simulink model "EV_system"  (R2022b)
settings: Solver=VariableStepAuto  StartTime=0.0  StopTime=10  RelTol=1e-3
libraries: fl_lib x45, nesl_utility x31, ee_lib x16, simulink x2, sdl_lib x1
(part 1 of 2)
settings Model: Creator=guenk  LastModifiedBy=user
settings DebuggingCC: UnitsInconsistencyMsg=none

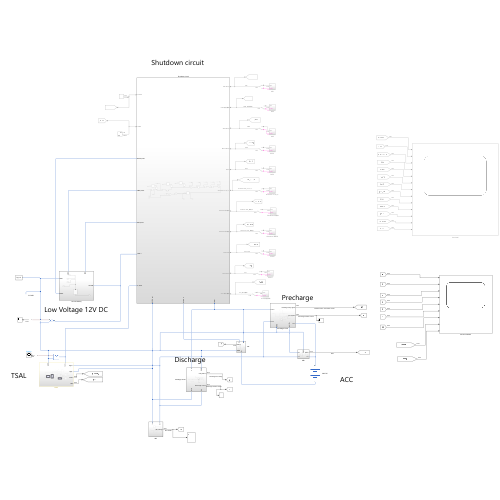
[thumbnail: Simulink's stored preview of the top-level diagram]
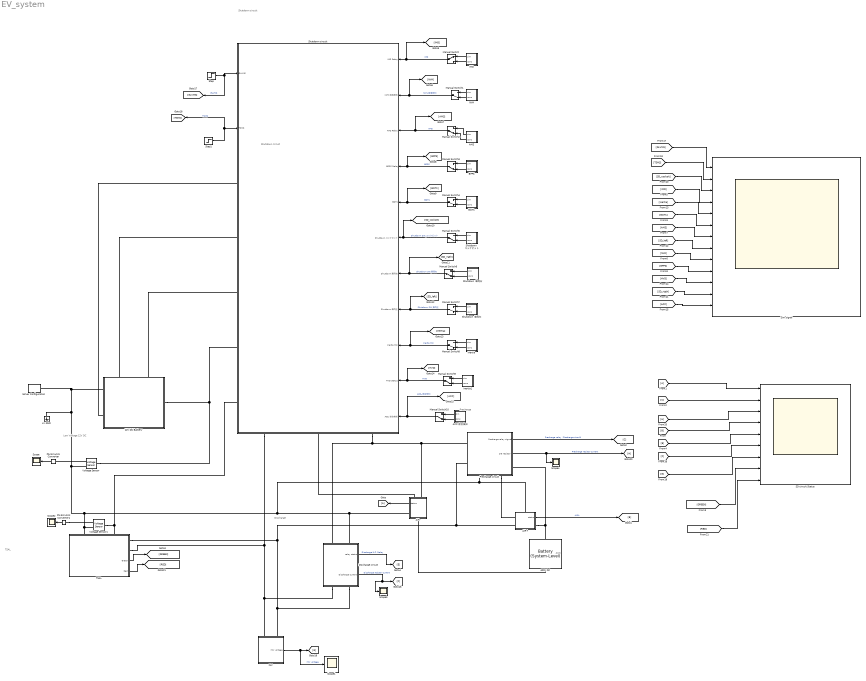
== system EV_system ==
  note: Precharge
  note: Discharge
  note: ACC
  note: Shutdown circuit
  note: Shutdown circuit
  note: Low Voltage 12V DC
  note: TSAL
  12V DC Battery : Subsystem
      settings: PortSchema="{\"entries\":[{\"content\":{\"sides\":[{\"content\":{\"connectorIds\":[\"LConn1\"]},\"type\":\"ConnectorPlacement.EquallySpacedRectSide\",\"uuid\":\"afe12baa-50eb-4c84-88de-44aa208358b8\"},{\"content\":{\"connectorIds\":[\"RConn1\",\"RConn2\"],\"side\":\"RIGHT\"},\"type\":\"ConnectorPlacement.EquallySpacedRectSide\",\"uuid\":\"76bb4b20-2fab-48ed-b43b-144bf9d425a6\"},{\"content\":{\"connectorIds\":[\"LConn2\",\"LConn3\"],\"side\":\"TOP\"},\"type\":\"ConnectorPlacement.EquallySpacedRectSide\",\"uuid\":\"9999fc27-06ad-4142-bc0d-dff183d80669\"},{\"content\":{\"connectorIds\":[],\"side\":\"BOTTOM\"},\"type\":\"ConnectorPlacement.EquallySpacedRectSide\",\"uuid\":\"0e91a3f8-fc00-4400-a4ba-be2b76be3e17\"}]},\"type\":\"ConnectorPlacement.EquallySpacedConnector\",\"uuid\":\"c30d57d7-3d09-4e60-950b-ccafea7457a0\"}],\"packageUris\":[\"http://schema.mathworks.com/mf0/Connector/R2020b\"],\"version\":\"1.0\"}"
  400V DC : sdl_lib/Sources/Battery (System-Level)  Vnom=400 V  R1=2 Ohm  prm_AH=sdl.enum.InfiniteFinite.Infinite  AH=50 A*hr  V1=11.5 V  AH1=25 A*hr  prm_R2=sdl.enum.DisabledEnabled.Disabled  R2=2000 Ohm  thermal_port=simscape.enum.thermaleffects.omit  thermal_mass=30000 J/K  i_specify=off  i_priority=None  i=0 A  i_nominal_specify=off  i_nominal_unit=A  i_nominal_value=1  v_specify=off  v_priority=None  v=0 V  v_nominal_specify=off  v_nominal_unit=V  v_nominal_value=1  charge_specify=off  charge_priority=High  charge=50 A*hr  charge_nominal_specify=off  charge_nominal_unit=A*hr  charge_nominal_value=1  temperature_specify=off  temperature_priority=High  temperature=300 K  temperature_nominal_specify=off  temperature_nominal_unit=K  temperature_nominal_value=1
      settings: InternalSimscapePortConfiguration="{\"Bottom\":[],\"Left\":[{\"id\":\"p\",\"label\":\"+\",\"type\":\"foundation.electrical.electrical\"}],\"Right\":[{\"id\":\"n\",\"label\":\"-\",\"type\":\"foundation.electrical.electrical\"}],\"Top\":[]}"
  ACC 嵌合検知 : Subsystem
  AIR+ : Subsystem
      settings: PortSchema="{\"entries\":[{\"content\":{\"sides\":[{\"content\":{\"connectorIds\":[\"LConn1\",\"LConn2\"]},\"type\":\"ConnectorPlacement.EquallySpacedRectSide\",\"uuid\":\"5e21f6f2-6e5b-4e9a-9905-27032e2692b4\"},{\"content\":{\"connectorIds\":[\"RConn1\",\"Out1\"],\"side\":\"RIGHT\"},\"type\":\"ConnectorPlacement.EquallySpacedRectSide\",\"uuid\":\"2e8b5de5-f94a-4975-8f74-9db9648a538a\"},{\"content\":{\"connectorIds\":[],\"side\":\"TOP\"},\"type\":\"ConnectorPlacement.EquallySpacedRectSide\",\"uuid\":\"84927b24-f1dd-4599-a8ed-fc9ccbdce19d\"},{\"content\":{\"connectorIds\":[\"RConn2\"],\"side\":\"BOTTOM\"},\"type\":\"ConnectorPlacement.EquallySpacedRectSide\",\"uuid\":\"5c556c2a-9a48-4544-808e-4306fc8b4db0\"}]},\"type\":\"ConnectorPlacement.EquallySpacedConnector\",\"uuid\":\"6bc14d99-2cc2-42ba-a5be-1190734add15\"}],\"packageUris\":[\"http://schema.mathworks.com/mf0/Connector/R2020b\"],\"version\":\"1.0\"}"
  AIR- : Subsystem
      settings: PortSchema="{\"entries\":[{\"content\":{\"sides\":[{\"content\":{\"connectorIds\":[\"LConn1\",\"LConn2\"]},\"type\":\"ConnectorPlacement.EquallySpacedRectSide\",\"uuid\":\"5e21f6f2-6e5b-4e9a-9905-27032e2692b4\"},{\"content\":{\"connectorIds\":[\"RConn1\"],\"side\":\"RIGHT\"},\"type\":\"ConnectorPlacement.EquallySpacedRectSide\",\"uuid\":\"2e8b5de5-f94a-4975-8f74-9db9648a538a\"},{\"content\":{\"connectorIds\":[],\"side\":\"TOP\"},\"type\":\"ConnectorPlacement.EquallySpacedRectSide\",\"uuid\":\"84927b24-f1dd-4599-a8ed-fc9ccbdce19d\"},{\"content\":{\"connectorIds\":[\"Out1\",\"RConn2\"],\"side\":\"BOTTOM\"},\"type\":\"ConnectorPlacement.EquallySpacedRectSide\",\"uuid\":\"3a3516dc-963b-428f-9da7-0a923f544841\"}]},\"type\":\"ConnectorPlacement.EquallySpacedConnector\",\"uuid\":\"6bc14d99-2cc2-42ba-a5be-1190734add15\"}],\"packageUris\":[\"http://schema.mathworks.com/mf0/Connector/R2020b\"],\"version\":\"1.0\"}"
  AMS : Subsystem
  BOTs : Subsystem
  BPPS : Subsystem
  Discharge circuit : Subsystem
      settings: PortSchema="{\"entries\":[{\"content\":{\"sides\":[{\"content\":{\"connectorIds\":[\"LConn1\",\"LConn2\"]},\"type\":\"ConnectorPlacement.EquallySpacedRectSide\",\"uuid\":\"f63f107d-6714-4216-92f5-cdaab8678b0a\"},{\"content\":{\"connectorIds\":[\"RConn1\",\"RConn2\"],\"side\":\"RIGHT\"},\"type\":\"ConnectorPlacement.EquallySpacedRectSide\",\"uuid\":\"52e9d350-d0e7-4a69-ac07-fd4c6d131c55\"},{\"content\":{\"connectorIds\":[],\"side\":\"TOP\"},\"type\":\"ConnectorPlacement.EquallySpacedRectSide\",\"uuid\":\"f71742c6-ae79-4014-be57-31d8cf50f3f5\"},{\"content\":{\"connectorIds\":[\"Out1\",\"Out2\"],\"side\":\"BOTTOM\"},\"type\":\"ConnectorPlacement.EquallySpacedRectSide\",\"uuid\":\"f82daf2f-c55b-4e43-8c2d-51f4f159019f\"}]},\"type\":\"ConnectorPlacement.EquallySpacedConnector\",\"uuid\":\"0630cc8e-bcff-4a39-a5b6-24d11d50336c\"}],\"packageUris\":[\"http://schema.mathworks.com/mf0/Connector/R2020b\"],\"version\":\"1.0\"}"
  From1 : From
  Goto : Goto
  IMD : Subsystem
  INV : Subsystem
      settings: PortSchema="{\"entries\":[{\"content\":{\"sides\":[{\"content\":{\"connectorIds\":[]},\"type\":\"ConnectorPlacement.EquallySpacedRectSide\",\"uuid\":\"e93b6f74-b762-4c41-b5e8-a2b4b8b47ac2\"},{\"content\":{\"connectorIds\":[\"Out1\"],\"side\":\"RIGHT\"},\"type\":\"ConnectorPlacement.EquallySpacedRectSide\",\"uuid\":\"b5ef1cd6-014c-4ca8-879d-b1281fc7d038\"},{\"content\":{\"connectorIds\":[\"LConn1\",\"LConn2\"],\"side\":\"TOP\"},\"type\":\"ConnectorPlacement.EquallySpacedRectSide\",\"uuid\":\"6817c51a-44f8-4b13-acb1-7166d3b3af9c\"}]},\"type\":\"ConnectorPlacement.EquallySpacedConnector\",\"uuid\":\"ca7f324f-d83d-4158-b69f-d878d7922f9c\"}],\"packageUris\":[\"http://schema.mathworks.com/mf0/Connector/R2020b\"],\"version\":\"1.0\"}"
  IWM : Subsystem
  Inertia : Subsystem
  Inertia1 : Subsystem
  LV GND : fl_lib/Electrical/Electrical Elements/Electrical Reference
  Manual Switch : ManualSwitch
  Manual Switch{1..10} (10 alike) : ManualSwitch  CurrentSetting=0
  PS-Simulink Converter : nesl_utility/PS-Simulink Converter  PhysicalDomain=network_engine_domain  SubClassName=ps_output  LeftPortType=input  RightPortType=output  PseudoPeriodic=off  Frequencies=[]  VectorFormat=inherit  Unit=inherit  AffineConversion=off
  PS-Simulink Converter1 : nesl_utility/PS-Simulink Converter  PhysicalDomain=network_engine_domain  SubClassName=ps_output  LeftPortType=input  RightPortType=output  PseudoPeriodic=off  Frequencies=[]  VectorFormat=inherit  Unit=inherit  AffineConversion=off
  Precharge circuit : Subsystem
      settings: PortSchema="{\"entries\":[{\"content\":{\"sides\":[{\"content\":{\"connectorIds\":[\"LConn1\",\"LConn2\"]},\"type\":\"ConnectorPlacement.EquallySpacedRectSide\",\"uuid\":\"e5d88cbf-b68f-42a2-978d-64f8ebea0f04\"},{\"content\":{\"connectorIds\":[\"Out1\",\"Out2\",\"RConn1\"],\"side\":\"RIGHT\"},\"type\":\"ConnectorPlacement.EquallySpacedRectSide\",\"uuid\":\"7cef2932-0641-450b-9147-52dafeed9344\"},{\"content\":{\"connectorIds\":[],\"side\":\"TOP\"},\"type\":\"ConnectorPlacement.EquallySpacedRectSide\",\"uuid\":\"11eb2363-e530-4ce9-8ad6-2747e1be63a1\"},{\"content\":{\"connectorIds\":[\"RConn2\",\"RConn3\"],\"side\":\"BOTTOM\"},\"type\":\"ConnectorPlacement.EquallySpacedRectSide\",\"uuid\":\"027fd163-b4b1-48ba-92c7-45894996ee1b\"}]},\"type\":\"ConnectorPlacement.EquallySpacedConnector\",\"uuid\":\"977f3c29-991d-4bcb-816f-8583683db08e\"}],\"packageUris\":[\"http://schema.mathworks.com/mf0/Connector/R2020b\"],\"version\":\"1.0\"}"
  SD circuit Status : Scope  NumInputPorts=9
  Scope{,1..4} (5 alike) : Scope
  Shutdown circuit : Subsystem
      settings: PortSchema="{\"entries\":[{\"content\":{\"sides\":[{\"content\":{\"connectorIds\":[\"In1\",\"In2\",\"LConn1\",\"LConn2\",\"LConn3\",\"LConn4\",\"LConn5\"]},\"type\":\"ConnectorPlacement.EquallySpacedRectSide\",\"uuid\":\"712c6cc5-6ca0-4be9-a23e-a688a1476752\"},{\"content\":{\"connectorIds\":[\"In3\",\"In4\",\"In5\",\"In6\",\"In7\",\"In8\",\"In9\",\"In10\",\"In11\",\"In12\",\"In13\"],\"side\":\"RIGHT\"},\"type\":\"ConnectorPlacement.EquallySpacedRectSide\",\"uuid\":\"0540c318-2f71-431c-925d-e4d2f84dd78c\"},{\"content\":{\"connectorIds\":[],\"side\":\"TOP\"},\"type\":\"ConnectorPlacement.EquallySpacedRectSide\",\"uuid\":\"244d453a-1328-4cec-905c-422ce983a29e\"},{\"content\":{\"connectorIds\":[\"RConn1\",\"RConn2\",\"RConn3\"],\"side\":\"BOTTOM\"},\"type\":\"ConnectorPlacement.EquallySpacedRectSide\",\"uuid\":\"22b99f56-0336-4f9d-80da-d662720265ed\"}]},\"type\":\"ConnectorPlacement.EquallySpacedConnector\",\"uuid\":\"1b5b4b2c-5218-4087-8834-57d2c09b23c8\"}],\"packageUris\":[\"http://schema.mathworks.com/mf0/Connector/R2020b\"],\"version\":\"1.0\"}"
  Shutdown コックピット : Subsystem
  Shutdown 車両右 : Subsystem
  Shutdown 車両左 : Subsystem
  Sim signal : Scope  NumInputPorts=13
  Solver Configuration : nesl_utility/Solver Configuration  PhysicalDomain=network_engine_domain  SubClassName=solver  LeftPortType=input  RightPortType=generic  Tones=[]  Harmonics=[]  SimulateNoise=off  Profile=off  UseLocalSampling=off  EnableSwitchedLinearOptims=on  FrequencyDomain=off  UseCCode=off  RelTol=0.001  AbsTol=0.001  MinStep=1e-09  ToWorkspace=off  RevertToSquareIcSolve=off  NumHomotopyIterations=100  PhasorMode=off  PhasorModeNumHarmonics=1  ConsistencySolver=NEWTON_XTOL_AFTER_FTOL  IndexReductionMethod=DerivativeReplacement  DoDC=on  ResidualTolerance=1e-09  ConsistencyTolSource=GLOBAL  ConsistencyAbsTol=0.001  ConsistencyRelTol=0.001  ConsistencyTolFactor=0.001  UseLocalSolver=off  LocalSolverChoice=NE_PARTITIONING_ADVANCER  ResolveIndetEquations=on  FunctionEvalNumThread=1  LocalSolverSampleTime=0.001  DoFixedCost=off  MaxNonlinIter=3  MaxModeIter=2  ComputeImpulses=off  ImpulseIterations=2  LinearAlgebra=auto  LinearAlgebraNumThread=0  EquationFormulation=NE_TIME_EF  DelaysMemoryBudget=1024  AutomaticFiltering=on  FilteringTimeConstant=0.001  PartitionStorageMethod=AS_NEEDED  PartitionMemoryBudget=1024  PartitionMethod=ROBUST
  Step : Step  SampleTime=0
  Step1 : Step  Time=2  SampleTime=0
  TSAL : Subsystem
      settings: PortSchema="{\"entries\":[{\"content\":{\"sides\":[{\"content\":{\"connectorIds\":[]},\"type\":\"ConnectorPlacement.EquallySpacedRectSide\",\"uuid\":\"5b688ee4-2581-4238-bfe6-47a5ea22367a\"},{\"content\":{\"connectorIds\":[\"RConn1\",\"RConn2\",\"Out1\",\"Out2\"],\"side\":\"RIGHT\"},\"type\":\"ConnectorPlacement.EquallySpacedRectSide\",\"uuid\":\"cfe53458-aa93-470c-96f6-0d5689e2c1e9\"},{\"content\":{\"connectorIds\":[\"LConn1\",\"LConn2\"],\"side\":\"TOP\"},\"type\":\"ConnectorPlacement.EquallySpacedRectSide\",\"uuid\":\"819ea1bd-7123-4be0-9b75-a399d2fff777\"},{\"content\":{\"connectorIds\":[],\"side\":\"BOTTOM\"},\"type\":\"ConnectorPlacement.EquallySpacedRectSide\",\"uuid\":\"3387471c-93ef-4528-ad06-c120c61af39c\"}]},\"type\":\"ConnectorPlacement.EquallySpacedConnector\",\"uuid\":\"02361df7-3d15-4a78-81f8-5caccd49837e\"}],\"packageUris\":[\"http://schema.mathworks.com/mf0/Connector/R2020b\"],\"version\":\"1.0\"}"
  Voltage Sensor : fl_lib/Electrical/Electrical Sensors/Voltage Sensor
  Voltage Sensor1 : fl_lib/Electrical/Electrical Sensors/Voltage Sensor
  wires:
  Step/1 -> [GLVMS], Shutdown circuit/1(GLVMS)  "GLVMS"
  IMD/1(sim) -> Manual Switch/1
  IMD/2(cons) -> Manual Switch/2
  Manual Switch/1 -> [IMD], Shutdown circuit/3(IMD Relay)  "IMD"
  Manual Switch1/1 -> Shutdown circuit/4(IWM 脱落検知), [IWM]  "IWM_脱落検知"
  IWM/2(cons) -> Manual Switch1/2
  IWM/1(sim) -> Manual Switch1/1
  AMS/1(sim) -> Manual Switch2/1
  AMS/2(cons) -> Manual Switch2/2
  Manual Switch2/1 -> [AMS], Shutdown circuit/5(AMS Relay)  "AMS"
  BPPS/2(cons) -> Manual Switch3/2
  BPPS/1(sim) -> Manual Switch3/1
  Manual Switch3/1 -> [BPPS], Shutdown circuit/6(BPPS Relay)  "BPPS"
  BOTs/1(sim) -> Manual Switch4/1
  BOTs/2(cons) -> Manual Switch4/2
  Manual Switch4/1 -> [BOTs], Shutdown circuit/7(BOTs)  "BOTs"
  Shutdown コックピット/2(cons) -> Manual Switch5/2
  Shutdown コックピット/1(sim) -> Manual Switch5/1
  Manual Switch5/1 -> Shutdown circuit/8(Shutdown コックピット), [SD_cockpit]  "Shutdown SW_コックピット"
  Shutdown 車両右/1(sim) -> Manual Switch6/1
  Shutdown 車両右/2(cons) -> Manual Switch6/2
  Manual Switch6/1 -> [SD_rigth], Shutdown circuit/9(Shutdown 車両右)  "Shutdown SW_車両右"
  Shutdown 車両左/2(cons) -> Manual Switch7/2
  Shutdown 車両左/1(sim) -> Manual Switch7/1
  Manual Switch7/1 -> Shutdown circuit/10(Shutdown 車両左), [SD_left]  "Shutdown SW_車両左"
  Inertia/1(sim) -> Manual Switch8/1
  Inertia/2(cons) -> Manual Switch8/2
  Manual Switch8/1 -> Shutdown circuit/11(Inertia SW), [Inertia]  "Inertia SW"
  Inertia1/2(cons) -> Manual Switch9/2
  Inertia1/1(sim) -> Manual Switch9/1
  Manual Switch9/1 -> [HVD], Shutdown circuit/12(HVD Status)  "HVD"
  ACC 嵌合検知/1(sim) -> Manual Switch10/1
  ACC 嵌合検知/2(cons) -> Manual Switch10/2
  Manual Switch10/1 -> [ACC], Shutdown circuit/13(ACC 嵌合検知)  "ACC_嵌合検知"
  Step1/1 -> [TSMS], Shutdown circuit/2(TSMS)  "TSMS"
  From1/1 -> SD circuit Status/1
  AIR-/1(status) -> Goto/1
  AIR+/1(status) -> [B]  "AIR+"
  [B] -> SD circuit Status/4
  [C] -> SD circuit Status/2
  Discharge circuit/1(relay status) -> [E]  "Discharge N.C. Relay"
  [E] -> SD circuit Status/5
  [IMD] -> Sim signal/4
  [IWM] -> Sim signal/9
  [AMS] -> Sim signal/7
  [BPPS] -> Sim signal/10
  [BOTs] -> Sim signal/6
  [SD_cockpit] -> Sim signal/3
  [SD_rigth] -> Sim signal/12
  [SD_left] -> Sim signal/8
  [Inertia] -> Sim signal/5
  [HVD] -> Sim signal/11
  [ACC] -> Sim signal/13
  [GLVMS] -> Sim signal/1
  [TSMS] -> Sim signal/2
  Precharge circuit/1(Precharge relay signal) -> [C]  "Precharge relay  (Precharge circuit)"
  Discharge circuit/2(Discharge current) -> Scope3/1, [F]  "Discharge resistor current"
  [F] -> SD circuit Status/6
  INV/1(INV voltage) -> Scope1/1, [G]  "INV voltage"
  [G] -> SD circuit Status/7
  Precharge circuit/2(pre resistor) -> Scope4/1, [H]  "Precharge resistor current"
  [H] -> SD circuit Status/3
  TSAL/1(Green) -> [GREEN]
  TSAL/2(Red) -> [RED]
  [GREEN] -> SD circuit Status/8
  [RED] -> SD circuit Status/9
  PS-Simulink Converter/1 -> Scope/1
  PS-Simulink Converter1/1 -> Scope2/1
  connections:
  12V DC Battery/LConn1 -- Voltage Sensor/LConn1 -- Shutdown circuit/LConn4
  12V DC Battery/LConn2 -- Shutdown circuit/LConn3
  12V DC Battery/LConn3 -- Shutdown circuit/LConn2
  12V DC Battery/RConn2 -- Shutdown circuit/LConn1
  Shutdown circuit/RConn3 -- Discharge circuit/LConn1 -- AIR-/LConn1 -- Precharge circuit/LConn1
  AIR-/RConn1 -- 400V DC/RConn1
  Precharge circuit/RConn3 -- AIR+/LConn2
  AIR-/LConn2 -- Shutdown circuit/RConn2
  Shutdown circuit/RConn1 -- INV/LConn1 -- Discharge circuit/RConn1 -- TSAL/RConn2
  Precharge circuit/LConn2 -- AIR+/LConn1 -- INV/LConn2 -- Discharge circuit/RConn2 -- TSAL/RConn1
  AIR+/RConn1 -- 400V DC/LConn1 -- Precharge circuit/RConn1
  Voltage Sensor/RConn1 -- PS-Simulink Converter/LConn1
  PS-Simulink Converter1/LConn1 -- Voltage Sensor1/RConn1
  Voltage Sensor1/LConn1 -- TSAL/LConn2 -- Shutdown circuit/LConn5
  Voltage Sensor1/RConn2 -- TSAL/LConn1 -- Voltage Sensor/RConn2 -- LV GND/LConn1 -- Solver Configuration/RConn1 -- 12V DC Battery/RConn1 -- AIR+/RConn2 -- Precharge circuit/RConn2 -- Discharge circuit/LConn2 -- AIR-/RConn2

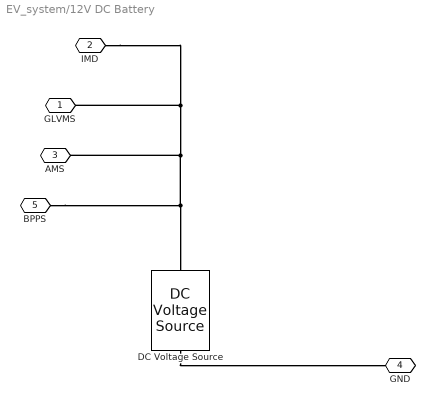
== system EV_system/12V DC Battery ==
  DC Voltage Source : fl_lib/Electrical/Electrical Sources/DC Voltage Source  v0=12 V
  GLVMS : PMIOPort  Side=Left
  IMD : PMIOPort  Port=2  Side=Left
  AMS : PMIOPort  Port=3  Side=Left
  GND : PMIOPort  Port=4  Side=Right
  BPPS : PMIOPort  Port=5  Side=Right
  connections:
  DC Voltage Source/RConn1 -- GND/RConn1
  IMD/RConn1 -- GLVMS/RConn1 -- BPPS/RConn1 -- DC Voltage Source/LConn1 -- AMS/RConn1

== system EV_system/ACC 嵌合検知 ==
  Constant : Constant
  Step1 : Step  Time=8  Before=1  After=0  SampleTime=0
  sim : Outport
  cons : Outport  Port=2
  wires:
  Constant/1 -> cons/1
  Step1/1 -> sim/1

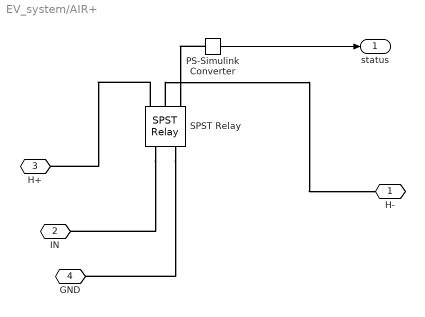
== system EV_system/AIR+ ==
  PS-Simulink Converter : nesl_utility/PS-Simulink Converter  PhysicalDomain=network_engine_domain  SubClassName=ps_output  LeftPortType=input  RightPortType=output  PseudoPeriodic=off  Frequencies=[]  VectorFormat=inherit  Unit=inherit  AffineConversion=off
  SPST Relay : ee_lib/Switches & Breakers/Relays/SPST Relay  block_choices=ee.enum.controlport.elec  R_closed=0.01 Ohm  G_open=1e-8 1/Ohm  Threshold=5  exposemeasurement=ee.enum.exposemeasurement.visible  V_rated=9 V  V_energize=75  V_deenergize=25  l_winding=0.08 H  r_winding=12.5 Ohm  g_winding=1e-9 1/Ohm  T_brk_C_S=3 ms  T_mak_C_S=6 ms  enable_faults=ee.enum.relays.enable.no  fault_action=ee.enum.relays.faultaction.none  fault_types=ee.enum.relays.faultTypes.winding  fault_condition_ps=ee.enum.relays.faultConditionSPSTps.csstuck  r_deg_closed_s=1e-9 Ohm  winding_tau_fault=1e-3 s  tau_fault=1e-3 s  enable_temporal_fault=ee.enum.relays.enable.no  t_fault_stick=1 s  t_fault_ComOpen=1 s  t_fault=1 s  enable_behavioral_fault=ee.enum.relays.enable.no  winding_max_permissible_voltage=inf V  n_fail_on_voltage=1  winding_max_permissible_current=inf A  max_permissible_current=inf A  t_fail_on_current=1 s
      settings: InternalSimscapePortConfiguration="{\"Bottom\":[],\"Left\":[{\"id\":\"p_winding\",\"label\":\"+\",\"type\":\"foundation.electrical.electrical\"},{\"id\":\"n_winding\",\"label\":\"-\",\"type\":\"foundation.electrical.electrical\"}],\"Right\":[{\"id\":\"S\",\"label\":\"S\",\"type\":\"foundation.electrical.electrical\"},{\"id\":\"COM\",\"label\":\"C\",\"type\":\"foundation.electrical.electrical\"},{\"id\":\"x\",\"label\":\"x\",\"type\":\"output\"}],\"Top\":[]}"
  H- : PMIOPort  Side=Left
  IN : PMIOPort  Port=2  Side=Left
  H+ : PMIOPort  Port=3  Side=Right
  GND : PMIOPort  Port=4  Side=Right
  status : Outport
  wires:
  PS-Simulink Converter/1 -> status/1
  connections:
  SPST Relay/RConn2 -- H-/RConn1
  SPST Relay/RConn1 -- H+/RConn1
  SPST Relay/LConn2 -- GND/RConn1
  SPST Relay/LConn1 -- IN/RConn1
  PS-Simulink Converter/LConn1 -- SPST Relay/RConn3

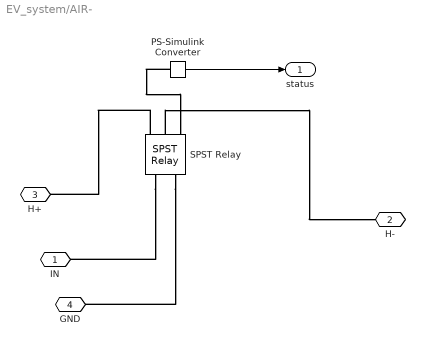
== system EV_system/AIR- ==
  PS-Simulink Converter : nesl_utility/PS-Simulink Converter  PhysicalDomain=network_engine_domain  SubClassName=ps_output  LeftPortType=input  RightPortType=output  PseudoPeriodic=off  Frequencies=[]  VectorFormat=inherit  Unit=inherit  AffineConversion=off
  SPST Relay : ee_lib/Switches & Breakers/Relays/SPST Relay  block_choices=ee.enum.controlport.elec  R_closed=0.01 Ohm  G_open=1e-8 1/Ohm  Threshold=5  exposemeasurement=ee.enum.exposemeasurement.visible  V_rated=9 V  V_energize=75  V_deenergize=25  l_winding=0.08 H  r_winding=12.5 Ohm  g_winding=1e-9 1/Ohm  T_brk_C_S=3 ms  T_mak_C_S=6 ms  enable_faults=ee.enum.relays.enable.no  fault_action=ee.enum.relays.faultaction.none  fault_types=ee.enum.relays.faultTypes.winding  fault_condition_ps=ee.enum.relays.faultConditionSPSTps.csstuck  r_deg_closed_s=1e-9 Ohm  winding_tau_fault=1e-3 s  tau_fault=1e-3 s  enable_temporal_fault=ee.enum.relays.enable.no  t_fault_stick=1 s  t_fault_ComOpen=1 s  t_fault=1 s  enable_behavioral_fault=ee.enum.relays.enable.no  winding_max_permissible_voltage=inf V  n_fail_on_voltage=1  winding_max_permissible_current=inf A  max_permissible_current=inf A  t_fail_on_current=1 s
      settings: InternalSimscapePortConfiguration="{\"Bottom\":[],\"Left\":[{\"id\":\"p_winding\",\"label\":\"+\",\"type\":\"foundation.electrical.electrical\"},{\"id\":\"n_winding\",\"label\":\"-\",\"type\":\"foundation.electrical.electrical\"}],\"Right\":[{\"id\":\"S\",\"label\":\"S\",\"type\":\"foundation.electrical.electrical\"},{\"id\":\"COM\",\"label\":\"C\",\"type\":\"foundation.electrical.electrical\"},{\"id\":\"x\",\"label\":\"x\",\"type\":\"output\"}],\"Top\":[]}"
  IN : PMIOPort  Side=Left
  H- : PMIOPort  Port=2  Side=Left
  H+ : PMIOPort  Port=3  Side=Right
  GND : PMIOPort  Port=4  Side=Right
  status : Outport
  wires:
  PS-Simulink Converter/1 -> status/1
  connections:
  SPST Relay/LConn1 -- IN/RConn1
  SPST Relay/LConn2 -- GND/RConn1
  SPST Relay/RConn1 -- H+/RConn1
  SPST Relay/RConn2 -- H-/RConn1
  PS-Simulink Converter/LConn1 -- SPST Relay/RConn3

== system EV_system/AMS ==
  Constant : Constant
  Step1 : Step  Time=12  Before=1  After=0  SampleTime=0
  sim : Outport
  cons : Outport  Port=2
  wires:
  Constant/1 -> cons/1
  Step1/1 -> sim/1

== system EV_system/BOTs ==
  Constant : Constant
  Step1 : Step  Time=6  Before=1  After=0  SampleTime=0
  sim : Outport
  cons : Outport  Port=2
  wires:
  Constant/1 -> cons/1
  Step1/1 -> sim/1

== system EV_system/BPPS ==
  Constant : Constant
  Step1 : Step  Time=14  Before=1  After=0  SampleTime=0
  sim : Outport
  cons : Outport  Port=2
  wires:
  Step1/1 -> sim/1
  Constant/1 -> cons/1

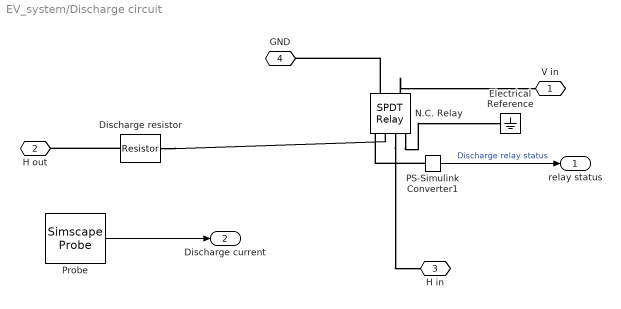
== system EV_system/Discharge circuit ==
  Discharge resistor : fl_lib/Electrical/Electrical Elements/Resistor  R=1500 Ohm  i_specify=off  i_priority=None  i=0 A  i_nominal_specify=off  i_nominal_unit=A  i_nominal_value=1  v_specify=off  v_priority=None  v=0 V  v_nominal_specify=off  v_nominal_unit=V  v_nominal_value=1
  Electrical Reference : fl_lib/Electrical/Electrical Elements/Electrical Reference
  N.C. Relay : ee_lib/Switches & Breakers/Relays/SPDT Relay  block_choices=ee.enum.controlport.elec  R_closed=0.01 Ohm  G_open=1e-8 1/Ohm  Threshold=0  exposemeasurement=ee.enum.exposemeasurement.visible  port_locations_spdt=ee.enum.relays.port_locations_spdt.standard  V_rated=9 V  V_energize=75  V_deenergize=25  l_winding=0.08 H  r_winding=12.5 Ohm  g_winding=1e-9 1/Ohm  T_brk_C_S1=0 s  T_mak_C_S1=0 s  T_brk_C_S2=0 s  T_mak_C_S2=0 s  enable_faults=ee.enum.relays.enable.no  fault_action=ee.enum.relays.faultaction.none  fault_types=ee.enum.relays.faultTypes.winding  fault_condition_ps=ee.enum.relays.faultConditionSPDTps.cs1stuck  r_deg_closed_s1=1e-9 Ohm  r_deg_closed_s2=1e-9 Ohm  winding_tau_fault=1e-3 s  tau_fault=1e-3 s  enable_temporal_fault=ee.enum.relays.enable.no  t_fault_stick=1 s  t_fault_ComOpen=1 s  t_fault=1 s  enable_behavioral_fault=ee.enum.relays.enable.no  winding_max_permissible_voltage=inf V  n_fail_on_voltage=1  winding_max_permissible_current=inf A  max_permissible_current=inf A  t_fail_on_current=1 s
      settings: InternalSimscapePortConfiguration="{\"Bottom\":[],\"Left\":[{\"id\":\"p_winding\",\"label\":\"+\",\"type\":\"foundation.electrical.electrical\"},{\"id\":\"n_winding\",\"label\":\"-\",\"type\":\"foundation.electrical.electrical\"}],\"Right\":[{\"id\":\"S2\",\"label\":\"S2\",\"type\":\"foundation.electrical.electrical\"},{\"id\":\"COM\",\"label\":\"C\",\"type\":\"foundation.electrical.electrical\"},{\"id\":\"S1\",\"label\":\"S1\",\"type\":\"foundation.electrical.electrical\"},{\"id\":\"x\",\"label\":\"x\",\"type\":\"output\"}],\"Top\":[]}"
  PS-Simulink Converter1 : nesl_utility/PS-Simulink Converter  PhysicalDomain=network_engine_domain  SubClassName=ps_output  LeftPortType=input  RightPortType=output  PseudoPeriodic=off  Frequencies=[]  VectorFormat=inherit  Unit=inherit  AffineConversion=off
  Probe : SimscapeProbe  BoundBlock=554  Variables={i}
  V in : PMIOPort  Side=Left
  H out : PMIOPort  Port=2  Side=Right
  H in : PMIOPort  Port=3  Side=Right
  GND : PMIOPort  Port=4  Side=Left
  relay status : Outport
  Discharge current : Outport  Port=2
  wires:
  PS-Simulink Converter1/1 -> relay status/1  "Discharge relay status"
  Probe/1 -> Discharge current/1
  connections:
  PS-Simulink Converter1/LConn1 -- N.C. Relay/RConn4
  N.C. Relay/LConn2 -- GND/RConn1
  N.C. Relay/RConn2 -- H in/RConn1
  Discharge resistor/RConn1 -- H out/RConn1
  Discharge resistor/LConn1 -- N.C. Relay/RConn3
  N.C. Relay/LConn1 -- V in/RConn1
  N.C. Relay/RConn1 -- Electrical Reference/LConn1

== system EV_system/IMD ==
  Constant : Constant
  Step1 : Step  Time=6  Before=1  After=0  SampleTime=0
  sim : Outport
  cons : Outport  Port=2
  wires:
  Constant/1 -> cons/1
  Step1/1 -> sim/1

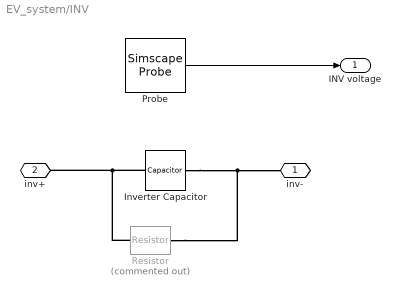
== system EV_system/INV ==
  Inverter Capacitor : fl_lib/Electrical/Electrical Elements/Capacitor  c=600 uF  r=1e-6 Ohm  g=0 1/Ohm  i_specify=off  i_priority=None  i=0 A  i_nominal_specify=off  i_nominal_unit=A  i_nominal_value=1  v_specify=off  v_priority=None  v=400 V  v_nominal_specify=off  v_nominal_unit=V  v_nominal_value=1  vc_specify=off  vc_priority=High  vc=400 V  vc_nominal_specify=off  vc_nominal_unit=V  vc_nominal_value=1
  Probe : SimscapeProbe  BoundBlock=543  Variables={vc}
  Resistor : fl_lib/Electrical/Electrical Elements/Resistor  Commented=on  R=191 kOhm  i_specify=off  i_priority=None  i=0 A  i_nominal_specify=off  i_nominal_unit=A  i_nominal_value=1  v_specify=off  v_priority=None  v=0 V  v_nominal_specify=off  v_nominal_unit=V  v_nominal_value=1
  inv- : PMIOPort  Side=Left
  inv+ : PMIOPort  Port=2  Side=Left
  INV voltage : Outport
  wires:
  Probe/1 -> INV voltage/1
  connections:
  Inverter Capacitor/RConn1 -- Resistor/RConn1 -- inv-/RConn1
  Inverter Capacitor/LConn1 -- Resistor/LConn1 -- inv+/RConn1

== system EV_system/IWM ==
  Constant : Constant
  Step1 : Step  Time=6  Before=1  After=0  SampleTime=0
  sim : Outport
  cons : Outport  Port=2
  wires:
  Step1/1 -> sim/1
  Constant/1 -> cons/1

== system EV_system/Inertia ==
  Constant : Constant
  Step1 : Step  Time=6  Before=1  After=0  SampleTime=0
  sim : Outport
  cons : Outport  Port=2
  wires:
  Constant/1 -> cons/1
  Step1/1 -> sim/1

== system EV_system/Inertia1 ==
  Constant : Constant
  Step1 : Step  Time=7  Before=1  After=0  SampleTime=0
  sim : Outport
  cons : Outport  Port=2
  wires:
  Step1/1 -> sim/1
  Constant/1 -> cons/1

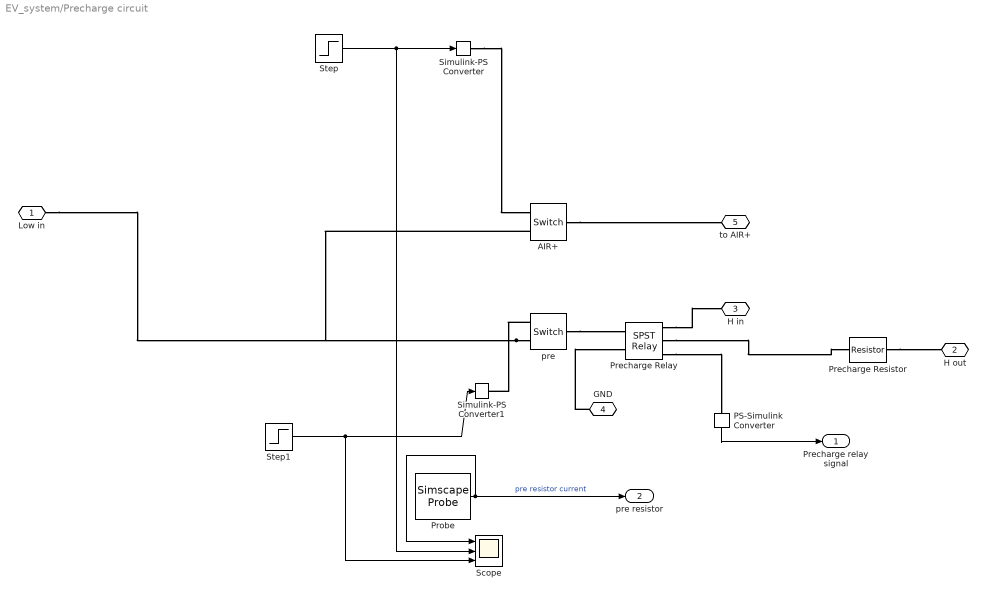
== system EV_system/Precharge circuit ==
  AIR+ : fl_lib/Electrical/Electrical Elements/Switch  R_closed=0.01 Ohm  G_open=1e-8 1/Ohm  Threshold=0.5  i_specify=off  i_priority=None  i=0 A  i_nominal_specify=off  i_nominal_unit=A  i_nominal_value=1  v_specify=off  v_priority=None  v=0 V  v_nominal_specify=off  v_nominal_unit=V  v_nominal_value=1
  PS-Simulink Converter : nesl_utility/PS-Simulink Converter  PhysicalDomain=network_engine_domain  SubClassName=ps_output  LeftPortType=input  RightPortType=output  PseudoPeriodic=off  Frequencies=[]  VectorFormat=inherit  Unit=inherit  AffineConversion=off
  Precharge Relay : ee_lib/Switches & Breakers/Relays/SPST Relay  block_choices=ee.enum.controlport.elec  R_closed=0.01 Ohm  G_open=1e-8 1/Ohm  Threshold=5  exposemeasurement=ee.enum.exposemeasurement.visible  V_rated=9 V  V_energize=75  V_deenergize=25  l_winding=0.08 H  r_winding=12.5 Ohm  g_winding=1e-9 1/Ohm  T_brk_C_S=6 ms  T_mak_C_S=3 ms  enable_faults=ee.enum.relays.enable.no  fault_action=ee.enum.relays.faultaction.none  fault_types=ee.enum.relays.faultTypes.winding  fault_condition_ps=ee.enum.relays.faultConditionSPSTps.csstuck  r_deg_closed_s=1e-9 Ohm  winding_tau_fault=1e-3 s  tau_fault=1e-3 s  enable_temporal_fault=ee.enum.relays.enable.no  t_fault_stick=1 s  t_fault_ComOpen=1 s  t_fault=1 s  enable_behavioral_fault=ee.enum.relays.enable.no  winding_max_permissible_voltage=inf V  n_fail_on_voltage=1  winding_max_permissible_current=inf A  max_permissible_current=inf A  t_fail_on_current=1 s
      settings: InternalSimscapePortConfiguration="{\"Bottom\":[],\"Left\":[{\"id\":\"p_winding\",\"label\":\"+\",\"type\":\"foundation.electrical.electrical\"},{\"id\":\"n_winding\",\"label\":\"-\",\"type\":\"foundation.electrical.electrical\"}],\"Right\":[{\"id\":\"S\",\"label\":\"S\",\"type\":\"foundation.electrical.electrical\"},{\"id\":\"COM\",\"label\":\"C\",\"type\":\"foundation.electrical.electrical\"},{\"id\":\"x\",\"label\":\"x\",\"type\":\"output\"}],\"Top\":[]}"
  Precharge Resistor : fl_lib/Electrical/Electrical Elements/Resistor  R=1 kOhm  i_specify=off  i_priority=None  i=0 A  i_nominal_specify=off  i_nominal_unit=A  i_nominal_value=1  v_specify=off  v_priority=None  v=0 V  v_nominal_specify=off  v_nominal_unit=V  v_nominal_value=1
  Probe : SimscapeProbe  BoundBlock=745  Variables={i}
  Scope : Scope  NumInputPorts=3
  Simulink-PS Converter : nesl_utility/Simulink-PS Converter  PhysicalDomain=network_engine_domain  SubClassName=ps_input  LeftPortType=input  RightPortType=output  PseudoPeriodic=off  Frequencies=[]  NoiseDistribution=none  NoiseParameters=[]  Unit=1  AffineConversion=off  FilteringAndDerivatives=provide  SimscapeFilterOrder=1  InputFilterTimeConstant=0.001  UdotUserProvided=0
  Simulink-PS Converter1 : nesl_utility/Simulink-PS Converter  PhysicalDomain=network_engine_domain  SubClassName=ps_input  LeftPortType=input  RightPortType=output  PseudoPeriodic=off  Frequencies=[]  NoiseDistribution=none  NoiseParameters=[]  Unit=1  AffineConversion=off  FilteringAndDerivatives=provide  SimscapeFilterOrder=1  InputFilterTimeConstant=0.001  UdotUserProvided=0
  Step : Step  Time=5.001  SampleTime=0
  Step1 : Step  Time=5  Before=1  After=0  SampleTime=0
  pre : fl_lib/Electrical/Electrical Elements/Switch  R_closed=0.01 Ohm  G_open=1e-8 1/Ohm  Threshold=0.5  i_specify=off  i_priority=None  i=0 A  i_nominal_specify=off  i_nominal_unit=A  i_nominal_value=1  v_specify=off  v_priority=None  v=0 V  v_nominal_specify=off  v_nominal_unit=V  v_nominal_value=1
  Low in : PMIOPort  Side=Left
  H out : PMIOPort  Port=2  Side=Left
  H in : PMIOPort  Port=3  Side=Right
  GND : PMIOPort  Port=4  Side=Right
  to AIR+ : PMIOPort  Port=5  Side=Right
  Precharge relay signal : Outport
  pre resistor : Outport  Port=2
  wires:
  Step1/1 -> Scope/3, Simulink-PS Converter1/1
  Step/1 -> Scope/2, Simulink-PS Converter/1
  Probe/1 -> Scope/1, pre resistor/1  "pre resistor current"
  PS-Simulink Converter/1 -> Precharge relay signal/1
  connections:
  Precharge Relay/RConn1 -- H in/RConn1
  AIR+/LConn1 -- to AIR+/RConn1
  pre/LConn1 -- Precharge Relay/LConn1
  GND/RConn1 -- Precharge Relay/LConn2
  Precharge Resistor/RConn1 -- H out/RConn1
  Simulink-PS Converter/RConn1 -- AIR+/RConn1
  pre/RConn1 -- Simulink-PS Converter1/RConn1
  Precharge Relay/RConn3 -- PS-Simulink Converter/LConn1
  Precharge Relay/RConn2 -- Precharge Resistor/LConn1
  pre/RConn2 -- Low in/RConn1 -- AIR+/RConn2

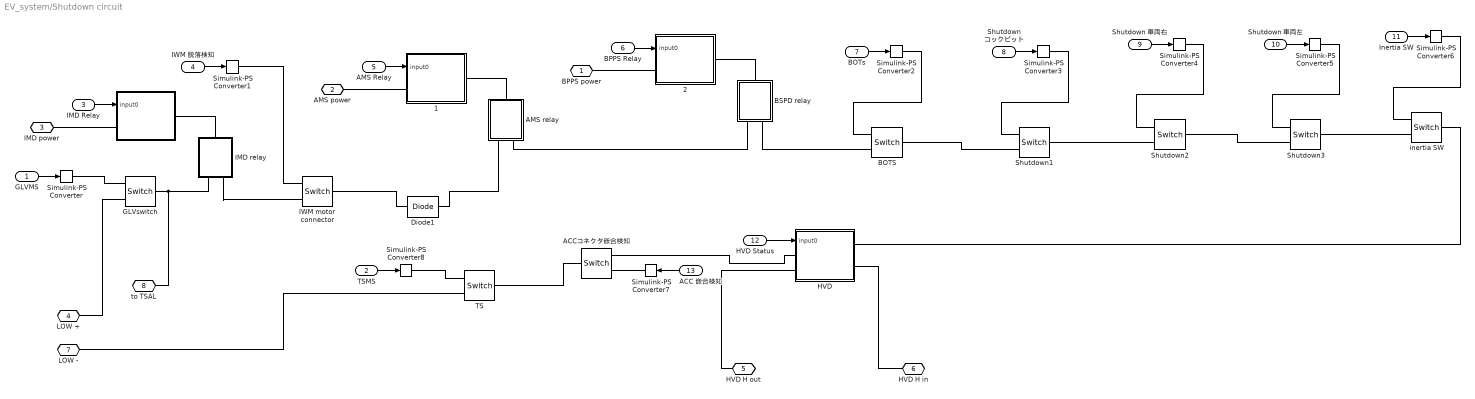
== system EV_system/Shutdown circuit ==
  GLVMS : Inport
  TSMS : Inport  Port=2
  IMD Relay : Inport  Port=3
  IWM 脱落検知 : Inport  Port=4
  AMS Relay : Inport  Port=5
  BPPS Relay : Inport  Port=6
  BOTs : Inport  Port=7
  Shutdown コックピット : Inport  Port=8
  Shutdown 車両右 : Inport  Port=9
  Shutdown 車両左 : Inport  Port=10
  Inertia SW : Inport  Port=11
  HVD Status : Inport  Port=12
  ACC 嵌合検知 : Inport  Port=13
  " " : Subsystem
  " 1" : Subsystem
  " 2" : Subsystem
  ACCコネクタ嵌合検知 : fl_lib/Electrical/Electrical Elements/Switch  R_closed=0.01 Ohm  G_open=1e-8 1/Ohm  Threshold=0.5  i_specify=off  i_priority=None  i=0 A  i_nominal_specify=off  i_nominal_unit=A  i_nominal_value=1  v_specify=off  v_priority=None  v=0 V  v_nominal_specify=off  v_nominal_unit=V  v_nominal_value=1
  AMS relay : Subsystem
  BOTS : fl_lib/Electrical/Electrical Elements/Switch  R_closed=0.01 Ohm  G_open=1e-8 1/Ohm  Threshold=0.5  i_specify=off  i_priority=None  i=0 A  i_nominal_specify=off  i_nominal_unit=A  i_nominal_value=1  v_specify=off  v_priority=None  v=0 V  v_nominal_specify=off  v_nominal_unit=V  v_nominal_value=1
  BSPD relay : Subsystem
  Diode1 : ee_lib/Semiconductors & Converters/Diode  ModelType=ee.enum.diode.modelType.pwl  TableType=ee.enum.diode.tableType.IfMat  IfMat=[.07, .12, .19, 1.75, 4.24, 7.32, 11.2; .16, .3, .72, 2.14, 5.02, 8.35, 13.12] A  VfMat=[.9, 1.15, 1.25, 1.5, 1.75, 2.17, 2.6, 2.85; .58, .68, .75, 1.1, 1.38, 1.77, 2.27, 2.7] V  TjVec=[25, 125] degC  VfVec=[.5, .7, .9, 1.3, 1.7, 2.1, 2.5] V  IfVec=[.1, .2, .5, 1, 2, 4, 7, 10] A  Vf=0.6 V  Ron=0.3 Ohm  Goff=1e-8 S  prmExp=ee.enum.diode.expParam.useTwo  I12=[.0137, .545] A  V12=[.6, .7] V  RS=0 Ohm  Tmeas=25 degC  IS=1e-12 A  ec=1  I1=0.0137 A  V1=0.6 V  N_series=1  N_parallel=1  Rz=0.3 Ohm  BV=inf V  C_param=ee.enum.diode.capParam.fixed  CJ=0 pF  CJ0=5 pF  Vvec=[.1, 10, 100] V  Cvec=[3.5, 1, .4] pF  VJ=1 V  Mgrad=0.5  FC=0.5  Q_param=ee.enum.diode.recoveryParam.off  iRM=-7.15 A  iF=4 A  didt=-750 A/us  trr_factor=3  trr=115 ns  Qrr=150 nA*s  Vr=-600 V  Ls=150 nH  Erec=0.03 J  TT=50 ns  tau=100 ns  T_param=ee.enum.diode.temperatureParam.off  Tdevice=25 degC  I1_T2=0.245 A  V1_T2=0.5 V  IS_T2=1.25e-7 A  Tmeas2=125 degC  XTI_param=ee.enum.diode.xtiParam.pn  XTI=3  EG_param=ee.enum.diode.egapParam.material_si  EG=1.11 eV  dBVdT=0 V/K  enable_faults=simscape.enum.onoff.off  fault_action=simscape.enum.assert.action.none  fault_types=ee.enum.diode.faults.open  tau_fault=1e-3 s  IfMat_faulted=[.07, .12, .19, 1.75, 4.24, 7.32, 11.2; .16, .3, .72, 2.14, 4.02, 6.35, 9.12] A  VfMat_faulted=[.9, 1.15, 1.25, 1.5, 1.75, 2.17, 2.6, 2.85; .58, .68, .75, 1.1, 1.38, 1.77, 2.27, 2.7] V  VfVec_faulted=[.5, .7, .9, 1.3, 1.7, 2.1, 2.5] V  IfVec_faulted=[.1, .2, .5, 1, 2, 4, 7, 10] A  Ropen_faulted=1000 Ohm  Gshort_faulted=1000 1/Ohm  Vf_faulted=0.6 V  Ron_faulted=0.3 Ohm  Goff_faulted=1e-8 S  I12_faulted=[.0137, .545] A  V12_faulted=[.6, .7] V  IS_faulted=1e-12 A  ec_faulted=1  I1_faulted=0.0137 A  V1_faulted=0.6 V  RS_faulted=0 Ohm  Rz_faulted=0.3 Ohm  BV_faulted=inf V  Cscale_faulted=100  enable_temporal_fault=simscape.enum.onoff.off  t_fault=inf s  enable_behavioral_fault=simscape.enum.onoff.off  max_permissible_voltage=inf V  n_fail_on_voltage=1  max_permissible_current=inf A  t_fail_on_current=1 s  max_permissible_dVdt=inf V/s  enable_fault_input=simscape.enum.onoff.off  i_specify=off  i_priority=None  i=0 A  i_nominal_specify=off  i_nominal_unit=A  i_nominal_value=1  v_specify=off  v_priority=None  v=0 V  v_nominal_specify=off  v_nominal_unit=V  v_nominal_value=1  v_capacitor_specify=off  v_capacitor_priority=None  v_capacitor=0 V  v_capacitor_nominal_specify=off  v_capacitor_nominal_unit=V  v_capacitor_nominal_value=1  i_diode_specify=off  i_diode_priority=None  i_diode=0 A  i_diode_nominal_specify=off  i_diode_nominal_unit=A  i_diode_nominal_value=1  v_diode_specify=off  v_diode_priority=None  v_diode=0 V  v_diode_nominal_specify=off  v_diode_nominal_unit=V  v_diode_nominal_value=1  i_capacitor_specify=off  i_capacitor_priority=None  i_capacitor=0 A  i_capacitor_nominal_specify=off  i_capacitor_nominal_unit=A  i_capacitor_nominal_value=1  power_dissipated_specify=off  power_dissipated_priority=None  power_dissipated=0 W  power_dissipated_nominal_specify=off  power_dissipated_nominal_unit=W  power_dissipated_nominal_value=1  fidelity_level=ee.enum.diode.fidelity.includeChargeDyn  rec_loss_model=ee.enum.diode.reverseRecoveryModel.fixed  ErecVal=0 J  ErecMat=zeros(2, 3) J  TjrecVec=[298.15, 398.15] K  IfrecVec=[.1, 1, 10] A  VrecVal=10 V  tFilter=1 / 1000 / 100 s  max_permissible_temperature=inf K  t_fail_on_temperature=1 s  thermal_network_parameterization=ee.enum.thermalNetworkTopology.junctionCase  Rth=[0, 10] K/W  Rth_Cauer=[1, 3, 10] K/W  Rth_Foster=[4, 6] K/W  thermal_mass_parameterization=ee.enum.thermalNetwork.timeconstant  thermal_mass=[0, 1] J/K  thermal_mass_Cauer=[.1, .3, 1] J/K  thermal_mass_Foster=[1.5, 3] J/K  thermal_time_constant=[0, 10] s  thermal_time_constant_Cauer=[1, 3, 10] s  thermal_time_constant_Foster=[6, 18] s  thermal_mass_initial_temperatures=[25, 25] degC  thermal_mass_initial_temperatures_Cauer=[25, 25, 25] degC  junction_thermal_mass=0.01 J/K  Tvec_initial_Foster=[25, 25, 25, 25] degC  no_thermal_network=0  junction_temperature_specify=off  junction_temperature_priority=None  junction_temperature=25 degC  junction_temperature_nominal_specify=off  junction_temperature_nominal_unit=degC  junction_temperature_nominal_value=1
  GLVswitch : fl_lib/Electrical/Electrical Elements/Switch  R_closed=0.01 Ohm  G_open=1e-8 1/Ohm  Threshold=0.5  i_specify=off  i_priority=None  i=0 A  i_nominal_specify=off  i_nominal_unit=A  i_nominal_value=1  v_specify=off  v_priority=None  v=0 V  v_nominal_specify=off  v_nominal_unit=V  v_nominal_value=1
  HVD : Subsystem
  IMD relay : Subsystem
  IWM motor connector : fl_lib/Electrical/Electrical Elements/Switch  R_closed=0.01 Ohm  G_open=1e-8 1/Ohm  Threshold=0.5  i_specify=off  i_priority=None  i=0 A  i_nominal_specify=off  i_nominal_unit=A  i_nominal_value=1  v_specify=off  v_priority=None  v=0 V  v_nominal_specify=off  v_nominal_unit=V  v_nominal_value=1
  Shutdown1 : fl_lib/Electrical/Electrical Elements/Switch  R_closed=0.01 Ohm  G_open=1e-8 1/Ohm  Threshold=0.5  i_specify=off  i_priority=None  i=0 A  i_nominal_specify=off  i_nominal_unit=A  i_nominal_value=1  v_specify=off  v_priority=None  v=0 V  v_nominal_specify=off  v_nominal_unit=V  v_nominal_value=1
  Shutdown2 : fl_lib/Electrical/Electrical Elements/Switch  R_closed=0.01 Ohm  G_open=1e-8 1/Ohm  Threshold=0.5  i_specify=off  i_priority=None  i=0 A  i_nominal_specify=off  i_nominal_unit=A  i_nominal_value=1  v_specify=off  v_priority=None  v=0 V  v_nominal_specify=off  v_nominal_unit=V  v_nominal_value=1
  Shutdown3 : fl_lib/Electrical/Electrical Elements/Switch  R_closed=0.01 Ohm  G_open=1e-8 1/Ohm  Threshold=0.5  i_specify=off  i_priority=None  i=0 A  i_nominal_specify=off  i_nominal_unit=A  i_nominal_value=1  v_specify=off  v_priority=None  v=0 V  v_nominal_specify=off  v_nominal_unit=V  v_nominal_value=1
  Simulink-PS Converter{,1..8} (9 alike) : nesl_utility/Simulink-PS Converter  PhysicalDomain=network_engine_domain  SubClassName=ps_input  LeftPortType=input  RightPortType=output  PseudoPeriodic=off  Frequencies=[]  NoiseDistribution=none  NoiseParameters=[]  Unit=1  AffineConversion=off  FilteringAndDerivatives=provide  SimscapeFilterOrder=1  InputFilterTimeConstant=0.001  UdotUserProvided=0
  TS : fl_lib/Electrical/Electrical Elements/Switch  R_closed=0.01 Ohm  G_open=1e-8 1/Ohm  Threshold=0.5  i_specify=off  i_priority=None  i=0 A  i_nominal_specify=off  i_nominal_unit=A  i_nominal_value=1  v_specify=off  v_priority=None  v=0 V  v_nominal_specify=off  v_nominal_unit=V  v_nominal_value=1
  inertia SW : fl_lib/Electrical/Electrical Elements/Switch  R_closed=0.01 Ohm  G_open=1e-8 1/Ohm  Threshold=0.5  i_specify=off  i_priority=None  i=0 A  i_nominal_specify=off  i_nominal_unit=A  i_nominal_value=1  v_specify=off  v_priority=None  v=0 V  v_nominal_specify=off  v_nominal_unit=V  v_nominal_value=1
  BPPS power : PMIOPort  Side=Left
  AMS power : PMIOPort  Port=2  Side=Left
  IMD power : PMIOPort  Port=3  Side=Left
  LOW + : PMIOPort  Port=4  Side=Left
  HVD H out : PMIOPort  Port=5  Side=Right
  HVD H in : PMIOPort  Port=6  Side=Right
  LOW - : PMIOPort  Port=7  Side=Right
  "to TSAL " : PMIOPort  Port=8  Side=Left
  wires:
  GLVMS/1 -> Simulink-PS Converter/1
  IMD Relay/1 -> " "/1(input0)
  IWM 脱落検知/1 -> Simulink-PS Converter1/1
  AMS Relay/1 -> " 1"/1(input0)
  BPPS Relay/1 -> " 2"/1(input0)
  BOTs/1 -> Simulink-PS Converter2/1
  Shutdown コックピット/1 -> Simulink-PS Converter3/1
  Shutdown 車両右/1 -> Simulink-PS Converter4/1
  Shutdown 車両左/1 -> Simulink-PS Converter5/1
  Inertia SW/1 -> Simulink-PS Converter6/1
  HVD Status/1 -> HVD/1(input0)
  ACC 嵌合検知/1 -> Simulink-PS Converter7/1
  TSMS/1 -> Simulink-PS Converter8/1
  connections:
  IMD power/RConn1 -- " "/LConn1
  LOW +/RConn1 -- GLVswitch/RConn2
  Simulink-PS Converter/RConn1 -- GLVswitch/RConn1
  IMD relay/RConn2 -- IWM motor connector/RConn2
  Simulink-PS Converter1/RConn1 -- IWM motor connector/RConn1
  " 1"/RConn1 -- AMS relay/LConn1
  AMS power/RConn1 -- " 1"/LConn1
  IWM motor connector/LConn1 -- Diode1/LConn1
  BPPS power/RConn1 -- " 2"/LConn1
  " 2"/RConn1 -- BSPD relay/LConn1
  BSPD relay/RConn1 -- AMS relay/RConn2
  BSPD relay/RConn2 -- BOTS/RConn2
  Simulink-PS Converter2/RConn1 -- BOTS/RConn1
  Simulink-PS Converter3/RConn1 -- Shutdown1/RConn1
  BOTS/LConn1 -- Shutdown1/RConn2
  Simulink-PS Converter4/RConn1 -- Shutdown2/RConn1
  Simulink-PS Converter5/RConn1 -- Shutdown3/RConn1
  Shutdown1/LConn1 -- Shutdown2/RConn2
  Shutdown2/LConn1 -- Shutdown3/RConn2
  Simulink-PS Converter6/RConn1 -- inertia SW/RConn1
  inertia SW/RConn2 -- Shutdown3/LConn1
  inertia SW/LConn1 -- HVD/RConn1
  HVD/RConn2 -- HVD H in/RConn1
  HVD/LConn2 -- HVD H out/RConn1
  HVD/LConn1 -- ACCコネクタ嵌合検知/RConn2
  ACCコネクタ嵌合検知/RConn1 -- Simulink-PS Converter7/RConn1
  Simulink-PS Converter8/RConn1 -- TS/RConn1
  ACCコネクタ嵌合検知/LConn1 -- TS/LConn1
  TS/RConn2 -- LOW -/RConn1
  " "/RConn1 -- IMD relay/LConn1
  GLVswitch/LConn1 -- IMD relay/RConn1 -- "to TSAL "/RConn1
  Diode1/RConn1 -- AMS relay/RConn1

== system EV_system/Shutdown コックピット ==
  Constant : Constant
  Step1 : Step  Time=10  Before=1  After=0  SampleTime=0
  sim : Outport
  cons : Outport  Port=2
  wires:
  Step1/1 -> sim/1
  Constant/1 -> cons/1

== system EV_system/Shutdown 車両右 ==
  Constant : Constant
  Step1 : Step  Time=6  Before=1  After=0  SampleTime=0
  sim : Outport
  cons : Outport  Port=2
  wires:
  Constant/1 -> cons/1
  Step1/1 -> sim/1

== system EV_system/Shutdown 車両左 ==
  Constant : Constant
  Step1 : Step  Time=6  Before=1  After=0  SampleTime=0
  sim : Outport
  cons : Outport  Port=2
  wires:
  Step1/1 -> sim/1
  Constant/1 -> cons/1
